simulink model "simulation_hovereye"  (R2020b)
settings: Solver=VariableStepAuto  StartTime=0.0  StopTime=30  RelTol=1e-3
values from neighbouring files (symbols this model uses):
  controlleur = struct('k1',0.5,                       'k2',2.1,                       'kf',1.0,                       'kn',2.4,                       'k_delta',7,                       'km',4.5,                       'kr',8.5                       )    [generateContolleur.m]    (also in run_hovereye.m = generateContolleur())
  drone = struct('MASS',               3.1,                      'J1',                 0.1,                     'J2',                 0.003,                     'G',                  9.81,                       'L',                  0.2,                  'epsilon',            -0.05                  )    [generatehovereye.m]    (also in run_hovereye.m = generatehovereye())
  omega_initial = [0; 0; 0]    [run_hovereye.m]
  p_initial = [0; 0; 0]    [run_hovereye.m]
  position_cible = [0.2; 0.2; 0.2]    [run_hovereye.m]
  q_initial = [0; 0; 0; 1]/sqrt(1)    [run_hovereye.m]
  v_initial = [0; 0; 0]    [run_hovereye.m]
libraries: sharedtransform x1
settings Model: Creator=florian  LastModifiedBy=florian

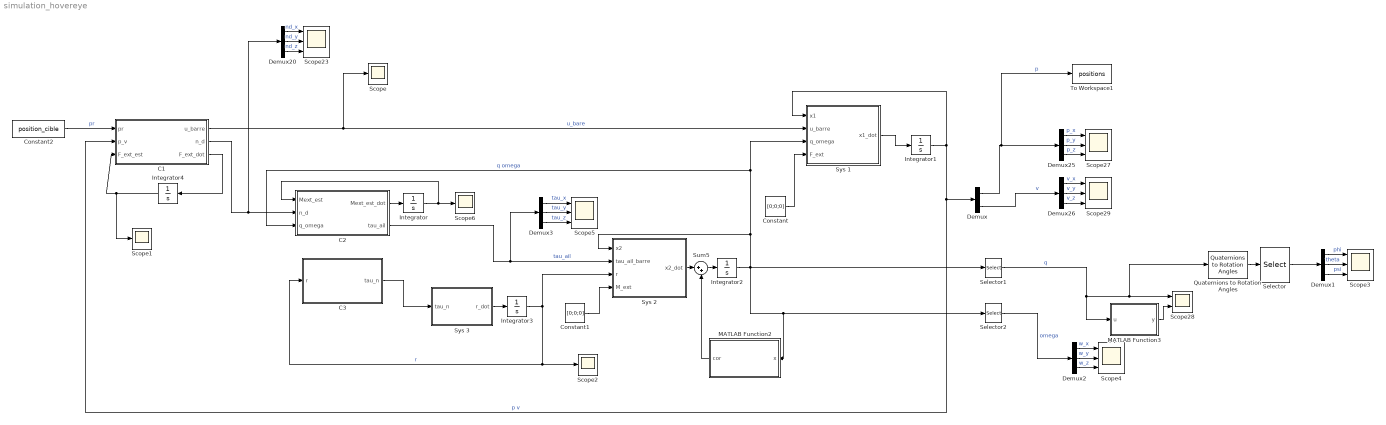
== system simulation_hovereye ==
  C1 : MATLAB Function  TreatAsAtomicUnit=on
  C2 : MATLAB Function  TreatAsAtomicUnit=on
  C3 : MATLAB Function  TreatAsAtomicUnit=on
  Constant : Constant  Value=[0;0;0]
  Constant1 : Constant  Value=[0;0;0]
  Constant2 : Constant  Value=position_cible
  Demux : Demux  Outputs=2
  Demux{1..3,20,25..26} (6 alike) : Demux  Outputs=3
  Integrator : Integrator
  Integrator1 : Integrator  InitialCondition=[p_initial; v_initial]
  Integrator2 : Integrator  InitialCondition=[q_initial; omega_initial]
  Integrator3 : Integrator
  Integrator4 : Integrator
  MATLAB Function2 : MATLAB Function  TreatAsAtomicUnit=on
  MATLAB Function3 : MATLAB Function  TreatAsAtomicUnit=on
  Quaternions to Rotation Angles : sharedtransform/Quaternions to Rotation Angles  rotationOrder=ZXY  aMode=aMode
      settings: SourceProductBaseCode=AE,PW,MT,UV,VE,VP
  Scope{,1..2,6} (4 alike) : Scope
  Scope{3..5,23,27,29} (6 alike) : Scope  NumInputPorts=3
  Scope28 : Scope  NumInputPorts=2
  Selector : Selector  InputPortWidth=3  IndexOptions=Index vector (dialog)  Indices=[2 3 1]  OutputSizes=1
  Selector1 : Selector  InputPortWidth=7  IndexOptions=Index vector (dialog)  Indices=[1:4]  OutputSizes=1
  Selector2 : Selector  InputPortWidth=7  IndexOptions=Index vector (dialog)  Indices=[5:7]  OutputSizes=1
  Sum5 : Sum  Inputs=|++
  Sys 1 : MATLAB Function  TreatAsAtomicUnit=on
  Sys 2 : MATLAB Function  TreatAsAtomicUnit=on
  Sys 3 : MATLAB Function  TreatAsAtomicUnit=on
  To Workspace1 : ToWorkspace  VariableName=positions  SampleTime=-1
  wires:
  Constant2/1 -> C1/1(pr)  "pr"
  C1/1(u_barre) -> Scope/1, Sys 1/2(u_barre)  "u_bare"
  C2/1(Mext_est_dot) -> Integrator/1
  Integrator/1 -> Scope6/1, C2/1(Mext_est)
  Sys 1/1(x1_dot) -> Integrator1/1
  Integrator1/1 -> Demux/1, C1/2(p_v), Sys 1/1(x1)  "p v"
  Constant/1 -> Sys 1/4(F_ext)
  Integrator2/1 -> Selector1/1, MATLAB Function2/1(x), Selector2/1, C2/3(q_omega), Sys 1/3(q_omega), Sys 2/1(x2)  "q omega"
  Sys 3/1(r_dot) -> Integrator3/1
  Integrator3/1 -> Sys 2/3(r), Scope2/1, C3/1(r)  "r"
  C3/1(tau_n) -> Sys 3/1(tau_n)
  Constant1/1 -> Sys 2/4(M_ext)
  C1/3(F_ext_dot) -> Integrator4/1
  Integrator4/1 -> Scope1/1, C1/3(F_ext_est)
  Demux20/1 -> Scope23/1  "nd_x"
  C1/2(n_d) -> Demux20/1, C2/2(n_d)
  Demux20/3 -> Scope23/3  "nd_z"
  Demux20/2 -> Scope23/2  "nd_y"
  Demux26/2 -> Scope29/2  "v_y"
  Demux26/1 -> Scope29/1  "v_x"
  Demux26/3 -> Scope29/3  "v_z"
  Demux25/2 -> Scope27/2  "p_y"
  Demux25/1 -> Scope27/1  "p_x"
  Demux25/3 -> Scope27/3  "p_z"
  Demux/2 -> Demux26/1  "v"
  Demux/1 -> To Workspace1/1, Demux25/1  "p"
  Selector1/1 -> MATLAB Function3/1(u), Quaternions to Rotation Angles/1, Scope28/1  "q"
  Selector/1 -> Demux1/1
  Demux1/2 -> Scope3/2  "theta"
  Demux1/3 -> Scope3/3  "psi"
  MATLAB Function3/1(y) -> Scope28/2
  Quaternions to Rotation Angles/1 -> Selector/1
  Demux1/1 -> Scope3/1  "phi"
  Selector2/1 -> Demux2/1  "omega"
  Demux2/3 -> Scope4/3  "w_z"
  Demux2/1 -> Scope4/1  "w_x"
  Demux2/2 -> Scope4/2  "w_y"
  C2/2(tau_ail) -> Demux3/1, Sys 2/2(tau_ail_barre)  "tau_ail"
  Demux3/1 -> Scope5/1  "tau_x"
  Demux3/2 -> Scope5/2  "tau_y"
  Demux3/3 -> Scope5/3  "tau_z"
  MATLAB Function2/1(cor) -> Sum5/2
  Sum5/1 -> Integrator2/1
  Sys 2/1(x2_dot) -> Sum5/1

== matlab function simulation_hovereye/C1 ==
  data: pr input; u_barre output; p_v input; F_ext_est input; n_d output size=3; controlleur parameter; drone parameter; F_ext_dot output
function [u_barre, n_d, F_ext_dot] = C1(pr, p_v, F_ext_est, controlleur, drone)
%#codegen
m = drone.MASS;
g = drone.G;
p = p_v(1:3);
v = p_v(4:6);

delta1 = p - pr;
delta2 = m*controlleur.k1*delta1 + m*v;

ubar_n = controlleur.k2 * delta2  + m*g*[0;0;1] + F_ext_est; %

u_barre = norm(ubar_n);
n_d = ubar_n/u_barre;
F_ext_dot = controlleur.kf*delta2;

== matlab function simulation_hovereye/Sys 1 ==
  data: x1 input; x1_dot output; u_barre input; q_omega input; F_ext input; drone parameter
function x1_dot = sys1(x1, u_barre, q_omega, F_ext,drone)
%#codegen
e3 = [0;0;1];
m = drone.MASS;
g = drone.G;

% xi = x1(1:3);
v = x1(4:6);

q = q_omega(1:4);
% omega = q_omega(5:7);

matrice_att = q2dcm(q);
xi_dot = v;
v_dot = [0;0;-g] + (1/m) * (u_barre * matrice_att * e3 + F_ext);

x1_dot = [xi_dot; v_dot];

== matlab function simulation_hovereye/C2 ==
  data: Mext_est input; Mext_est_dot output size=3; n_d input; q_omega input; tau_ail output; controlleur parameter; drone parameter
function [Mext_est_dot, tau_ail] = C2(Mext_est, n_d, q_omega, controlleur, drone)
%#codegen

e3 = [0;0;1];

q = q_omega(1:4);
omega = q_omega(5:7);

matrice_att = q2dcm(q);
eta = matrice_att' * n_d;

delta = omega - controlleur.kn*cross(e3, eta);

tau_ail = -controlleur.k_delta * delta  + cross(e3, eta) - controlleur.kn*drone.J1*cross(cross(e3, omega), eta)- cross(e3, (matrice_att' * Mext_est)); %
Mext_est_dot = controlleur.km * matrice_att * cross(delta, e3);

== matlab function simulation_hovereye/Sys 2 ==
  data: x2 input; x2_dot output; tau_ail_barre input; r input; M_ext input; drone parameter
function x2_dot = sys2(x2, tau_ail_barre, r, M_ext, drone)
%#codegen
e3 = [0;0;1];

q = x2(1:4);
omega = x2(5:7);

matrice_att = q2dcm(q);

q_dot = 0.5*quat_product([0;omega],q);
omega_dot = (1/drone.J1) * (drone.J2 - drone.J1)* r* cross(e3, omega) + tau_ail_barre + cross(e3, matrice_att'*M_ext);

x2_dot = [q_dot; omega_dot];

== matlab function simulation_hovereye/C3 ==
  data: r input; tau_n output; controlleur parameter; drone parameter
function tau_n = C3(r, controlleur, drone)
%#codegen

tau_n = - drone.J2 * controlleur.kr * r;

== matlab function simulation_hovereye/Sys 3 ==
  data: r_dot output; tau_n input; drone parameter
function r_dot = sys3( tau_n, drone)

r_dot = tau_n / drone.J2;

== matlab function simulation_hovereye/MATLAB Function2 ==
  data: x input; cor output
function cor  = fcn(x)
%#codegen
q  = x(1:4);
n = norm(q);
mismatch = 1-n;
cor = [mismatch*q; 0;0;0;];

== matlab function simulation_hovereye/MATLAB Function3 ==
  data: u input; y output
function y = fcn(u)
%#codegen

y = norm(u);
